simulink model "z1_a"  (R2021a)
settings: Solver=VariableStepAuto  StartTime=0.0  StopTime=10.0  RelTol=1e-3
settings Model: Creator=48604  LastModifiedBy=48604

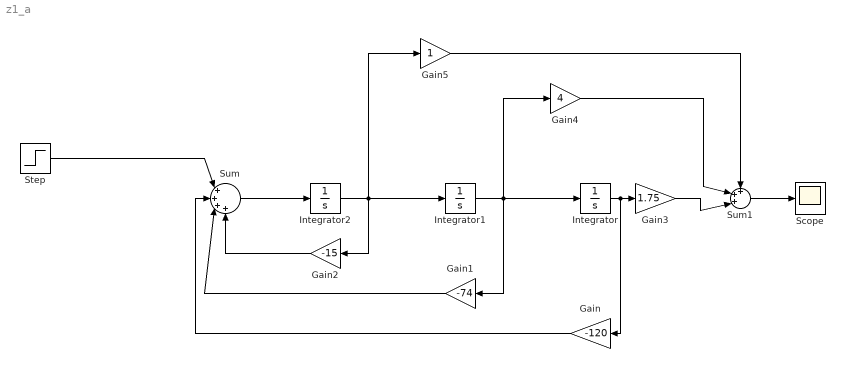
== system z1_a ==
  Gain : Gain  Gain=-120
  Gain1 : Gain  Gain=-74
  Gain2 : Gain  Gain=-15
  Gain3 : Gain  Gain=1.75
  Gain4 : Gain  Gain=4
  Gain5 : Gain
  Integrator : Integrator
  Integrator1 : Integrator
  Integrator2 : Integrator
  Scope : Scope
  Step : Step  SampleTime=1
  Sum : Sum  Inputs=|++++
  Sum1 : Sum  Inputs=+++|
  wires:
  Integrator/1 -> Gain/1, Gain3/1
  Gain3/1 -> Sum1/3
  Integrator1/1 -> Integrator/1, Gain1/1, Gain4/1
  Integrator2/1 -> Integrator1/1, Gain2/1, Gain5/1
  Sum/1 -> Integrator2/1
  Step/1 -> Sum/1
  Gain5/1 -> Sum1/1
  Gain4/1 -> Sum1/2
  Sum1/1 -> Scope/1
  Gain2/1 -> Sum/4
  Gain1/1 -> Sum/3
  Gain/1 -> Sum/2
